simulink model "ModiOmkar_19EE30018_model"  (R2017a)
settings: Solver=FixedStepAuto  StartTime=0.0  StopTime=0.08  FixedStep=1e-7  MaxStep=1e-7  RelTol=1e-6
libraries: powerlib x162, powerlib_meascontrol x12, simulink x12
(part 1 of 2)
settings Model: Creator=Triptendu  LastModifiedBy=HP
settings SFSimCC: SimUseLocalCustomCode=on
settings RTWCC: RTWUseLocalCustomCode=on

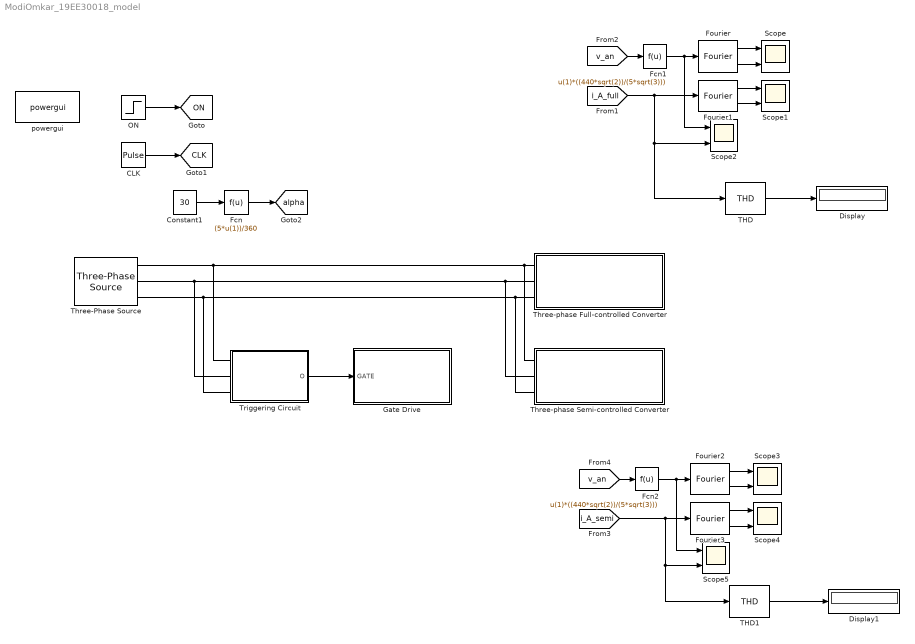
== system ModiOmkar_19EE30018_model ==
  CLK : DiscretePulseGenerator  PulseType=Time based  Period=40e-6  PulseWidth=50
  Constant1 : Constant  Value=30
  Display : Display
  Display1 : Display
  Fcn : Fcn  Expr=(5*u(1))/360
  Fcn1 : Fcn  Expr=u(1)*((440*sqrt(2))/(5*sqrt(3)))
  Fcn2 : Fcn  Expr=u(1)*((440*sqrt(2))/(5*sqrt(3)))
  Fourier{,1..3} (4 alike) : powerlib_meascontrol/Measurements/Fourier  Freq=50  n=1  InInit=[0, 0]  Ts=1e-6
  Gate Drive : Subsystem
  ON : Step  Time=0.002  SampleTime=0
  Scope{,1..5} (6 alike) : Scope  NumInputPorts=2
  THD : powerlib_meascontrol/Measurements/THD  Freq=50  Ts=0
  THD1 : powerlib_meascontrol/Measurements/THD  Freq=50  Ts=0
  Three-Phase Source : powerlib/Electrical Sources/Three-Phase Source  InternalConnection=Y  VoltagePhases=off  Voltage=440  PhaseAngle=0  Voltage_phases=[25e3 25e3 25e3]/sqrt(3)  PhaseAngles_phases=[0 -120 +120]  Frequency=50  NonIdealSource=on  SpecifyImpedance=off  Resistance=0  Inductance=0  ShortCircuitLevel=100e6  BaseVoltage=440  XRratio=7  BusType=swing  Pref=10e3  Qref=0  Prefabc=[10e3, 10e3, 10e3]  Qrefabc=[0, 0, 0]  Qmin=-inf  Qmax=inf
  Three-phase Full-controlled Converter : Subsystem
  Three-phase Semi-controlled Converter : Subsystem
  Triggering Circuit : Subsystem
  powergui : powerlib/powergui  Priority=1  SimulationMode=Discrete  SampleTime=1e-7  frequency=60  Iterations=50  frequencyindice=0  Pbase=100e6  ErrMax=1e-4  UnitsV=kV  UnitsW=MW  buscounter=0  FunctionMessages=off  echomessages=off  EnableUseOfTLC=off  CurrentSourceSwitches=off  DisableSnubberDevices=off  DisableRonSwitches=off  DisableVfSwitches=off  DisplayEquations=off  AutomaticDiscreteSolvers=off  SolverType=Backward Euler  Interpol=off  ExternalGateDelay=off  methode=off  Ts=100  x0status=blocks  SPID=on  SwTol=0  HookPort=off  NonlinearTolerance=1e-4  nMaxIteration=100  ContinueOnMaxIteration=off  RestoreLinks=warning  ResistiveCurrentMeasurement=off  Frange=[0:2:500]  Ylog=off  Xlog=on  ShowGrid=off  save=off  variable=ZData  structure=i_ABC_semi  ZoomFFT=on  StartTime=0.04  cycles=2  DisplayStyle=2  fundamental=50  FreqAxis=off  MaxFrequency=1000  frequencyindicesteady=1  RmsSteady=1  display=off
  tag scope: CLK=global, ON=global, alpha=global
  wires:
  ON/1 -> [ON]
  CLK/1 -> [CLK]
  Constant1/1 -> Fcn/1
  Fcn/1 -> [alpha]
  Triggering Circuit/1(O) -> Gate Drive/1(GATE)
  [i_A_full] -> Scope2/2, THD/1, Fourier1/1
  Fourier/1 -> Scope/1
  Fourier1/1 -> Scope1/1
  [v_an] -> Fcn1/1
  Fcn1/1 -> Scope2/1, Fourier/1
  Fourier/2 -> Scope/2
  Fourier1/2 -> Scope1/2
  [i_A_semi] -> Fourier3/1, THD1/1, Scope5/2
  Fourier2/1 -> Scope3/1
  [v_an] -> Fcn2/1
  Fcn2/1 -> Scope5/1, Fourier2/1
  Fourier3/1 -> Scope4/1
  Fourier2/2 -> Scope3/2
  Fourier3/2 -> Scope4/2
  THD/1 -> Display/1
  THD1/1 -> Display1/1
  connections:
  Triggering Circuit/LConn1 -- Three-phase Semi-controlled Converter/LConn1 -- Three-phase Full-controlled Converter/LConn1 -- Three-Phase Source/RConn1
  Triggering Circuit/LConn2 -- Three-phase Full-controlled Converter/LConn2 -- Three-phase Semi-controlled Converter/LConn2 -- Three-Phase Source/RConn2
  Triggering Circuit/LConn3 -- Three-phase Full-controlled Converter/LConn3 -- Three-phase Semi-controlled Converter/LConn3 -- Three-Phase Source/RConn3

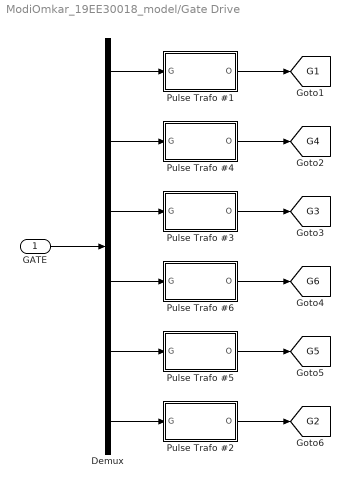
== system ModiOmkar_19EE30018_model/Gate Drive ==
  GATE : Inport
  Demux : Demux  Outputs=6
  Pulse Trafo #1 : Subsystem
  Pulse Trafo #2 : Subsystem
  Pulse Trafo #3 : Subsystem
  Pulse Trafo #4 : Subsystem
  Pulse Trafo #5 : Subsystem
  Pulse Trafo #6 : Subsystem
  tag scope: G1=global, G2=global, G3=global, G4=global, G5=global, G6=global
  wires:
  Demux/6 -> Pulse Trafo #2/1(G)
  Demux/5 -> Pulse Trafo #5/1(G)
  Demux/4 -> Pulse Trafo #6/1(G)
  Demux/3 -> Pulse Trafo #3/1(G)
  Demux/2 -> Pulse Trafo #4/1(G)
  Demux/1 -> Pulse Trafo #1/1(G)
  GATE/1 -> Demux/1
  Pulse Trafo #1/1(O) -> [G1]
  Pulse Trafo #4/1(O) -> [G4]
  Pulse Trafo #3/1(O) -> [G3]
  Pulse Trafo #6/1(O) -> [G6]
  Pulse Trafo #5/1(O) -> [G5]
  Pulse Trafo #2/1(O) -> [G2]

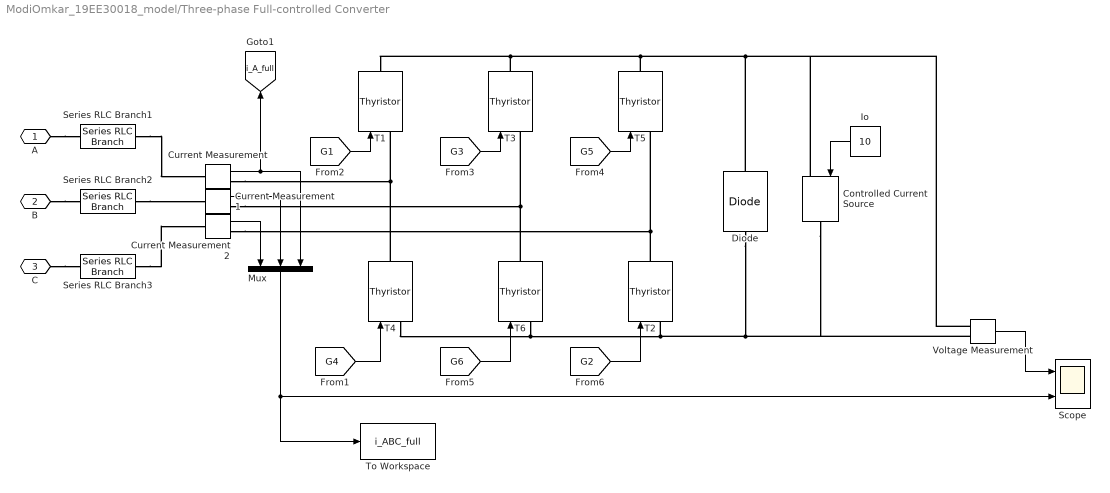
== system ModiOmkar_19EE30018_model/Three-phase Full-controlled Converter ==
  Controlled Current Source : powerlib/Electrical Sources/Controlled Current Source  Initialize=off  Source_Type=DC  Amplitude=0  Phase=0  Frequency=0  Measurements=None
  Current Measurement : powerlib/Measurements/Current Measurement  PhasorSimulation=off  OutputType=Complex  PSBequivalent=0
  Current Measurement1 : powerlib/Measurements/Current Measurement  PhasorSimulation=off  OutputType=Complex  PSBequivalent=0
  Current Measurement2 : powerlib/Measurements/Current Measurement  PhasorSimulation=off  OutputType=Complex  PSBequivalent=0
  Diode : powerlib/Power Electronics/Diode  Ron=1e-6  Lon=0  Vf=0  IC=0  UseSnubber=0  Rs=1e12  Cs=0  Measurements=off
  Io : Constant  Value=10
  Mux : Mux  Inputs=3
  Scope : Scope  NumInputPorts=2
  Series RLC Branch1 : powerlib/Elements/Series RLC Branch  LConnTagsString=__new0  RConnTagsString=__new0  BranchType=R  Resistance=1e-3  Inductance=5e-3  SetiL0=off  InitialCurrent=0  Capacitance=1e-6  Setx0=off  InitialVoltage=0  Measurements=None
  Series RLC Branch2 : powerlib/Elements/Series RLC Branch  LConnTagsString=__new0  RConnTagsString=__new0  BranchType=R  Resistance=1e-3  Inductance=5e-3  SetiL0=off  InitialCurrent=0  Capacitance=1e-6  Setx0=off  InitialVoltage=0  Measurements=None
  Series RLC Branch3 : powerlib/Elements/Series RLC Branch  LConnTagsString=__new0  RConnTagsString=__new0  BranchType=R  Resistance=1e-3  Inductance=5e-3  SetiL0=off  InitialCurrent=0  Capacitance=1e-6  Setx0=off  InitialVoltage=0  Measurements=None
  T{1..6} (6 alike) : powerlib/Power Electronics/Thyristor  Ron=1e-3  Lon=0  Vf=0  IC=0  Rs=1e12  Cs=inf  Measurements=off
  To Workspace : ToWorkspace  VariableName=i_ABC_full  SaveFormat=Structure With Time  SampleTime=-1
  Voltage Measurement : powerlib/Measurements/Voltage Measurement  PhasorSimulation=off  OutputType=Complex  PSBequivalent=0
  A : PMIOPort  Side=Left
  B : PMIOPort  Port=2  Side=Left
  C : PMIOPort  Port=3  Side=Left
  tag scope: i_A_full=global
  wires:
  [G6] -> T6/1
  [G2] -> T2/1
  [G4] -> T4/1
  [G5] -> T5/1
  [G3] -> T3/1
  [G1] -> T1/1
  Voltage Measurement/1 -> Scope/1
  Current Measurement/1 -> Mux/3, [i_A_full]
  Current Measurement1/1 -> Mux/2
  Current Measurement2/1 -> Mux/1
  Io/1 -> Controlled Current Source/1
  Mux/1 -> To Workspace/1, Scope/2
  connections:
  T2/RConn1 -- Current Measurement2/RConn1 -- T5/LConn1
  T5/RConn1 -- Voltage Measurement/LConn1 -- Controlled Current Source/LConn1 -- Diode/RConn1 -- T3/RConn1 -- T1/RConn1
  T6/RConn1 -- Current Measurement1/RConn1 -- T3/LConn1
  T4/RConn1 -- Current Measurement/RConn1 -- T1/LConn1
  C/RConn1 -- Series RLC Branch3/RConn1
  Series RLC Branch1/LConn1 -- Current Measurement/LConn1
  B/RConn1 -- Series RLC Branch2/RConn1
  T4/LConn1 -- T6/LConn1 -- Voltage Measurement/LConn2 -- Controlled Current Source/RConn1 -- Diode/LConn1 -- T2/LConn1
  A/RConn1 -- Series RLC Branch1/RConn1
  Series RLC Branch2/LConn1 -- Current Measurement1/LConn1
  Series RLC Branch3/LConn1 -- Current Measurement2/LConn1

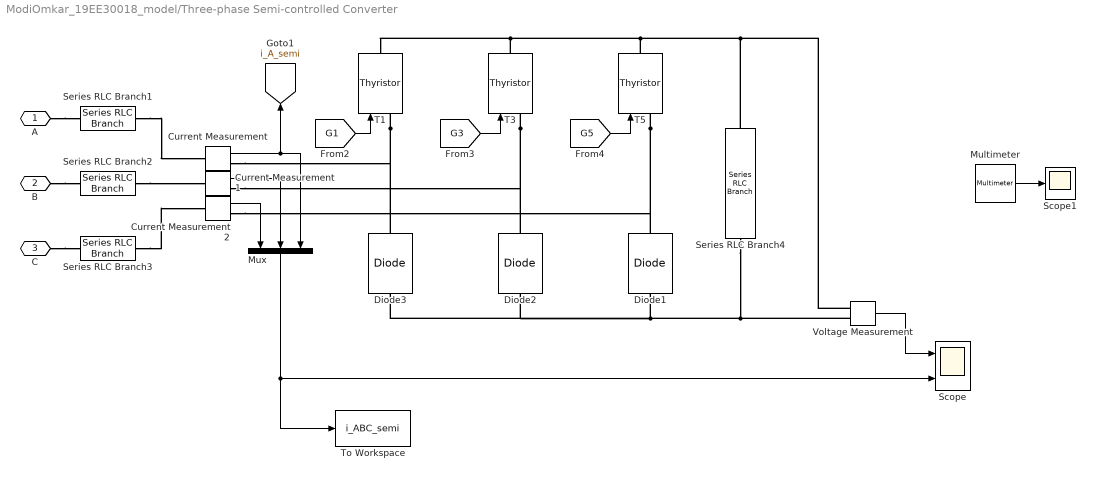
== system ModiOmkar_19EE30018_model/Three-phase Semi-controlled Converter ==
  Current Measurement : powerlib/Measurements/Current Measurement  PhasorSimulation=off  OutputType=Complex  PSBequivalent=0
  Current Measurement1 : powerlib/Measurements/Current Measurement  PhasorSimulation=off  OutputType=Complex  PSBequivalent=0
  Current Measurement2 : powerlib/Measurements/Current Measurement  PhasorSimulation=off  OutputType=Complex  PSBequivalent=0
  Diode1 : powerlib/Power Electronics/Diode  Ron=1e-3  Lon=0  Vf=0  IC=0  UseSnubber=0  Rs=1e12  Cs=inf  Measurements=off
  Diode2 : powerlib/Power Electronics/Diode  Ron=1e-3  Lon=0  Vf=0  IC=0  UseSnubber=0  Rs=1e12  Cs=inf  Measurements=off
  Diode3 : powerlib/Power Electronics/Diode  Ron=1e-3  Lon=0  Vf=0  IC=0  UseSnubber=0  Rs=1e12  Cs=inf  Measurements=off
  Multimeter : powerlib/Measurements/Multimeter  PhasorSimulation=off  OutputType=Complex  sel=1  L=1  Gain=1  yselected={'Ib: Three-phase Semi-controlled Converter/Series RLC Branch4'};  PSBOutputType=1  PSBequivalent=0  AxesSetting=[0,0.1,-100,100]  Display=0  SavedBlockNames=-11
  Mux : Mux  Inputs=3
  Scope : Scope  NumInputPorts=2
  Scope1 : Scope
  Series RLC Branch1 : powerlib/Elements/Series RLC Branch  LConnTagsString=__new0  RConnTagsString=__new0  BranchType=R  Resistance=1e-3  Inductance=5e-3  SetiL0=off  InitialCurrent=0  Capacitance=1e-6  Setx0=off  InitialVoltage=0  Measurements=None
  Series RLC Branch2 : powerlib/Elements/Series RLC Branch  LConnTagsString=__new0  RConnTagsString=__new0  BranchType=R  Resistance=1e-3  Inductance=5e-3  SetiL0=off  InitialCurrent=0  Capacitance=1e-6  Setx0=off  InitialVoltage=0  Measurements=None
  Series RLC Branch3 : powerlib/Elements/Series RLC Branch  LConnTagsString=__new0  RConnTagsString=__new0  BranchType=R  Resistance=1e-3  Inductance=5e-3  SetiL0=off  InitialCurrent=0  Capacitance=1e-6  Setx0=off  InitialVoltage=0  Measurements=None
  Series RLC Branch4 : powerlib/Elements/Series RLC Branch  LConnTagsString=__new0  RConnTagsString=__new0  BranchType=RL  Resistance=50.7188  Inductance=100e-3  SetiL0=off  InitialCurrent=0  Capacitance=1e-6  Setx0=off  InitialVoltage=0  Measurements=Branch current
  T1 : powerlib/Power Electronics/Thyristor  Ron=1e-3  Lon=0  Vf=0  IC=0  Rs=1e12  Cs=inf  Measurements=off
  T3 : powerlib/Power Electronics/Thyristor  Ron=1e-3  Lon=0  Vf=0  IC=0  Rs=1e12  Cs=inf  Measurements=off
  T5 : powerlib/Power Electronics/Thyristor  Ron=1e-3  Lon=0  Vf=0  IC=0  Rs=1e12  Cs=inf  Measurements=off
  To Workspace : ToWorkspace  VariableName=i_ABC_semi  SaveFormat=Structure With Time  SampleTime=-1
  Voltage Measurement : powerlib/Measurements/Voltage Measurement  PhasorSimulation=off  OutputType=Complex  PSBequivalent=0
  A : PMIOPort  Side=Left
  B : PMIOPort  Port=2  Side=Left
  C : PMIOPort  Port=3  Side=Left
  tag scope: i_A_semi=global
  wires:
  Current Measurement2/1 -> Mux/1
  Current Measurement1/1 -> Mux/2
  Current Measurement/1 -> [i_A_semi], Mux/3
  Voltage Measurement/1 -> Scope/1
  [G1] -> T1/1
  [G3] -> T3/1
  [G5] -> T5/1
  Multimeter/1 -> Scope1/1
  Mux/1 -> To Workspace/1, Scope/2
  connections:
  Series RLC Branch3/LConn1 -- Current Measurement2/LConn1
  Series RLC Branch2/LConn1 -- Current Measurement1/LConn1
  A/RConn1 -- Series RLC Branch1/RConn1
  Voltage Measurement/LConn2 -- Series RLC Branch4/LConn1 -- Diode2/LConn1 -- Diode3/LConn1 -- Diode1/LConn1
  B/RConn1 -- Series RLC Branch2/RConn1
  Series RLC Branch1/LConn1 -- Current Measurement/LConn1
  C/RConn1 -- Series RLC Branch3/RConn1
  T1/LConn1 -- Diode3/RConn1 -- Current Measurement/RConn1
  T3/LConn1 -- Diode2/RConn1 -- Current Measurement1/RConn1
  Voltage Measurement/LConn1 -- Series RLC Branch4/RConn1 -- T1/RConn1 -- T3/RConn1 -- T5/RConn1
  T5/LConn1 -- Diode1/RConn1 -- Current Measurement2/RConn1

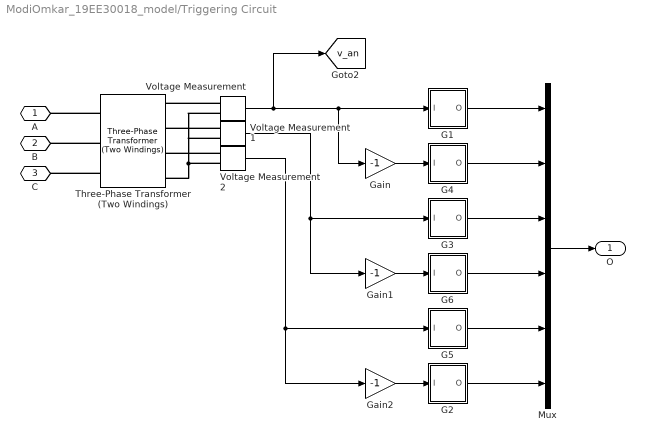
== system ModiOmkar_19EE30018_model/Triggering Circuit ==
  G1 : Subsystem
  G2 : Subsystem
  G3 : Subsystem
  G4 : Subsystem
  G5 : Subsystem
  G6 : Subsystem
  Gain : Gain  Gain=-1
  Gain1 : Gain  Gain=-1
  Gain2 : Gain  Gain=-1
  Mux : Mux  Inputs=6
  Three-Phase Transformer (Two Windings) : powerlib/Elements/Three-Phase Transformer (Two Windings)  Winding1Connection=Y  Winding2Connection=Yn  CoreType=Three single-phase transformers  SetSaturation=off  Hysteresis=off  DataFile='hysteresis'  SetInitialFlux=off  Measurements=None  UNITS=SI  NominalPower=[ 100 , 50 ]  Winding1=[440*sqrt(2) 0 0]  Winding2=[5*sqrt(3) 0 0]  Rm=1e6  Lm=1e6  L0=0.5  Saturation=[0 0;0.00044536 1.3723;0.18557 1.7382]  InitialFluxes=[ 0.8 , -0.8 , 0.7 ]  BreakLoop=off  DiscreteSolver=Trapezoidal iterative  DataType=on  TransfoNumber=1
  Voltage Measurement : powerlib/Measurements/Voltage Measurement  PhasorSimulation=off  OutputType=Complex  PSBequivalent=0
  Voltage Measurement1 : powerlib/Measurements/Voltage Measurement  PhasorSimulation=off  OutputType=Complex  PSBequivalent=0
  Voltage Measurement2 : powerlib/Measurements/Voltage Measurement  PhasorSimulation=off  OutputType=Complex  PSBequivalent=0
  A : PMIOPort  Side=Left
  B : PMIOPort  Port=2  Side=Left
  C : PMIOPort  Port=3  Side=Left
  O : Outport
  tag scope: v_an=global
  wires:
  G1/1(O) -> Mux/1
  Gain/1 -> G4/1(I)
  Gain1/1 -> G6/1(I)
  G5/1(O) -> Mux/5
  Voltage Measurement1/1 -> G3/1(I), Gain1/1
  Voltage Measurement2/1 -> G5/1(I), Gain2/1
  Gain2/1 -> G2/1(I)
  Voltage Measurement/1 -> [v_an], G1/1(I), Gain/1
  G3/1(O) -> Mux/3
  G4/1(O) -> Mux/2
  G2/1(O) -> Mux/6
  G6/1(O) -> Mux/4
  Mux/1 -> O/1
  connections:
  Voltage Measurement2/LConn2 -- Voltage Measurement1/LConn2 -- Voltage Measurement/LConn2 -- Three-Phase Transformer (Two Windings)/RConn4
  Voltage Measurement2/LConn1 -- Three-Phase Transformer (Two Windings)/RConn3
  Voltage Measurement/LConn1 -- Three-Phase Transformer (Two Windings)/RConn1
  Three-Phase Transformer (Two Windings)/LConn2 -- B/RConn1
  Voltage Measurement1/LConn1 -- Three-Phase Transformer (Two Windings)/RConn2
  Three-Phase Transformer (Two Windings)/LConn1 -- A/RConn1
  Three-Phase Transformer (Two Windings)/LConn3 -- C/RConn1

== system ModiOmkar_19EE30018_model/Gate Drive/Pulse Trafo #1 ==
  G : Inport
  D1 : powerlib/Power Electronics/Diode  Ron=0.001  Lon=0  Vf=0.7  IC=0  UseSnubber=off  Rs=inf  Cs=0  Measurements=off
  Ground5 : powerlib/Elements/Ground  LConnTagsString=a
  Ground6 : powerlib/Elements/Ground  LConnTagsString=a
  Mosfet : powerlib/Power Electronics/Mosfet  Ron=0.1  Lon=0  Rd=0.01  Vfd=0  IC=0  Rs=1e5  Cs=inf  Measurements=off
  R : powerlib/Elements/Series RLC Branch  LConnTagsString=__new0  RConnTagsString=__new0  BranchType=R  Resistance=10  Inductance=60e-3  SetiL0=off  InitialCurrent=0  Capacitance=1e-6  Setx0=off  InitialVoltage=0  Measurements=None
  R (for simulation) : powerlib/Elements/Series RLC Branch  LConnTagsString=__new0  RConnTagsString=__new0  BranchType=R  Resistance=1e6  Inductance=60e-3  SetiL0=off  InitialCurrent=0  Capacitance=1e-6  Setx0=off  InitialVoltage=0  Measurements=None
  Subsystem : Subsystem
  Vcc : powerlib/Electrical Sources/DC Voltage Source  Amplitude=20  Measurements=None
  Zener Diode : Subsystem  mask(Zener Diode){Vz=40, Rzt=10, Rzk=400, Izm=5, Vf=0.7, Ron=1e-3}
      mask prompts: Vz "Zener Voltage Vz (V)"; Rzt "Dynamic Impedance Zzt (ohms)"; Rzk "Knee Impedance Zzk (ohms)"; Izm "Maximum Continuous Current Izm (A)"; Vf "Forward Voltage Drop Vf (V)"; Ron "On Resistance Ron (ohms)"
      mask help:
      | Implements a zener diode block.
      | Use values from standard datasheets to populate block dialog
  pulse transformer : powerlib/Elements/Linear Transformer  UNITS=SI  NominalPower=[0.5 500e3 ]  winding1=[20 0.08 2e-6]  winding2=[20 0.08 2e-6]  ThreeWindings=off  winding3=[5 0.8 20e-6]  RmLm=[400 5e-3]  Measurements=None  DataType=on
  O : Outport
  wires:
  Subsystem/1(O) -> O/1
  G/1 -> Mosfet/1
  connections:
  Subsystem/LConn2 -- pulse transformer/RConn2
  pulse transformer/RConn1 -- Subsystem/LConn1
  D1/LConn1 -- Zener Diode/RConn1 -- R (for simulation)/RConn1
  D1/RConn1 -- Vcc/RConn1 -- R/LConn1
  Ground5/LConn1 -- Vcc/LConn1
  Ground6/LConn1 -- Mosfet/RConn1
  Mosfet/LConn1 -- Zener Diode/LConn1 -- R (for simulation)/LConn1 -- pulse transformer/LConn2
  R/RConn1 -- pulse transformer/LConn1

== system ModiOmkar_19EE30018_model/Gate Drive/Pulse Trafo #2 ==
  G : Inport
  D1 : powerlib/Power Electronics/Diode  Ron=0.001  Lon=0  Vf=0.7  IC=0  UseSnubber=off  Rs=inf  Cs=0  Measurements=off
  Ground5 : powerlib/Elements/Ground  LConnTagsString=a
  Ground6 : powerlib/Elements/Ground  LConnTagsString=a
  Mosfet : powerlib/Power Electronics/Mosfet  Ron=0.1  Lon=0  Rd=0.01  Vfd=0  IC=0  Rs=1e5  Cs=inf  Measurements=off
  R : powerlib/Elements/Series RLC Branch  LConnTagsString=__new0  RConnTagsString=__new0  BranchType=R  Resistance=10  Inductance=60e-3  SetiL0=off  InitialCurrent=0  Capacitance=1e-6  Setx0=off  InitialVoltage=0  Measurements=None
  R (for simulation) : powerlib/Elements/Series RLC Branch  LConnTagsString=__new0  RConnTagsString=__new0  BranchType=R  Resistance=1e6  Inductance=60e-3  SetiL0=off  InitialCurrent=0  Capacitance=1e-6  Setx0=off  InitialVoltage=0  Measurements=None
  Subsystem : Subsystem
  Vcc : powerlib/Electrical Sources/DC Voltage Source  Amplitude=20  Measurements=None
  Zener Diode : Subsystem  mask(Zener Diode){Vz=40, Rzt=10, Rzk=400, Izm=5, Vf=0.7, Ron=1e-3}
      mask prompts: Vz "Zener Voltage Vz (V)"; Rzt "Dynamic Impedance Zzt (ohms)"; Rzk "Knee Impedance Zzk (ohms)"; Izm "Maximum Continuous Current Izm (A)"; Vf "Forward Voltage Drop Vf (V)"; Ron "On Resistance Ron (ohms)"
      mask help:
      | Implements a zener diode block.
      | Use values from standard datasheets to populate block dialog
  pulse transformer : powerlib/Elements/Linear Transformer  UNITS=SI  NominalPower=[0.5 500e3 ]  winding1=[20 0.08 2e-6]  winding2=[20 0.08 2e-6]  ThreeWindings=off  winding3=[5 0.8 20e-6]  RmLm=[400 5e-3]  Measurements=None  DataType=on
  O : Outport
  wires:
  G/1 -> Mosfet/1
  Subsystem/1(O) -> O/1
  connections:
  R/RConn1 -- pulse transformer/LConn1
  pulse transformer/LConn2 -- R (for simulation)/LConn1 -- Zener Diode/LConn1 -- Mosfet/LConn1
  Ground6/LConn1 -- Mosfet/RConn1
  Ground5/LConn1 -- Vcc/LConn1
  Vcc/RConn1 -- R/LConn1 -- D1/RConn1
  R (for simulation)/RConn1 -- Zener Diode/RConn1 -- D1/LConn1
  pulse transformer/RConn1 -- Subsystem/LConn1
  Subsystem/LConn2 -- pulse transformer/RConn2

== system ModiOmkar_19EE30018_model/Gate Drive/Pulse Trafo #3 ==
  G : Inport
  D1 : powerlib/Power Electronics/Diode  Ron=0.001  Lon=0  Vf=0.7  IC=0  UseSnubber=off  Rs=inf  Cs=0  Measurements=off
  Ground5 : powerlib/Elements/Ground  LConnTagsString=a
  Ground6 : powerlib/Elements/Ground  LConnTagsString=a
  Mosfet : powerlib/Power Electronics/Mosfet  Ron=0.1  Lon=0  Rd=0.01  Vfd=0  IC=0  Rs=1e5  Cs=inf  Measurements=off
  R : powerlib/Elements/Series RLC Branch  LConnTagsString=__new0  RConnTagsString=__new0  BranchType=R  Resistance=10  Inductance=60e-3  SetiL0=off  InitialCurrent=0  Capacitance=1e-6  Setx0=off  InitialVoltage=0  Measurements=None
  R (for simulation) : powerlib/Elements/Series RLC Branch  LConnTagsString=__new0  RConnTagsString=__new0  BranchType=R  Resistance=1e6  Inductance=60e-3  SetiL0=off  InitialCurrent=0  Capacitance=1e-6  Setx0=off  InitialVoltage=0  Measurements=None
  Subsystem : Subsystem
  Vcc : powerlib/Electrical Sources/DC Voltage Source  Amplitude=20  Measurements=None
  Zener Diode : Subsystem  mask(Zener Diode){Vz=40, Rzt=10, Rzk=400, Izm=5, Vf=0.7, Ron=1e-3}
      mask prompts: Vz "Zener Voltage Vz (V)"; Rzt "Dynamic Impedance Zzt (ohms)"; Rzk "Knee Impedance Zzk (ohms)"; Izm "Maximum Continuous Current Izm (A)"; Vf "Forward Voltage Drop Vf (V)"; Ron "On Resistance Ron (ohms)"
      mask help:
      | Implements a zener diode block.
      | Use values from standard datasheets to populate block dialog
  pulse transformer : powerlib/Elements/Linear Transformer  UNITS=SI  NominalPower=[0.5 500e3 ]  winding1=[20 0.08 2e-6]  winding2=[20 0.08 2e-6]  ThreeWindings=off  winding3=[5 0.8 20e-6]  RmLm=[400 5e-3]  Measurements=None  DataType=on
  O : Outport
  wires:
  Subsystem/1(O) -> O/1
  G/1 -> Mosfet/1
  connections:
  Subsystem/LConn2 -- pulse transformer/RConn2
  pulse transformer/RConn1 -- Subsystem/LConn1
  D1/LConn1 -- Zener Diode/RConn1 -- R (for simulation)/RConn1
  D1/RConn1 -- R/LConn1 -- Vcc/RConn1
  Ground5/LConn1 -- Vcc/LConn1
  Ground6/LConn1 -- Mosfet/RConn1
  Mosfet/LConn1 -- Zener Diode/LConn1 -- R (for simulation)/LConn1 -- pulse transformer/LConn2
  R/RConn1 -- pulse transformer/LConn1

== system ModiOmkar_19EE30018_model/Gate Drive/Pulse Trafo #4 ==
  G : Inport
  D1 : powerlib/Power Electronics/Diode  Ron=0.001  Lon=0  Vf=0.7  IC=0  UseSnubber=off  Rs=inf  Cs=0  Measurements=off
  Ground5 : powerlib/Elements/Ground  LConnTagsString=a
  Ground6 : powerlib/Elements/Ground  LConnTagsString=a
  Mosfet : powerlib/Power Electronics/Mosfet  Ron=0.1  Lon=0  Rd=0.01  Vfd=0  IC=0  Rs=1e5  Cs=inf  Measurements=off
  R : powerlib/Elements/Series RLC Branch  LConnTagsString=__new0  RConnTagsString=__new0  BranchType=R  Resistance=10  Inductance=60e-3  SetiL0=off  InitialCurrent=0  Capacitance=1e-6  Setx0=off  InitialVoltage=0  Measurements=None
  R (for simulation) : powerlib/Elements/Series RLC Branch  LConnTagsString=__new0  RConnTagsString=__new0  BranchType=R  Resistance=1e6  Inductance=60e-3  SetiL0=off  InitialCurrent=0  Capacitance=1e-6  Setx0=off  InitialVoltage=0  Measurements=None
  Subsystem : Subsystem
  Vcc : powerlib/Electrical Sources/DC Voltage Source  Amplitude=20  Measurements=None
  Zener Diode : Subsystem  mask(Zener Diode){Vz=40, Rzt=10, Rzk=400, Izm=5, Vf=0.7, Ron=1e-3}
      mask prompts: Vz "Zener Voltage Vz (V)"; Rzt "Dynamic Impedance Zzt (ohms)"; Rzk "Knee Impedance Zzk (ohms)"; Izm "Maximum Continuous Current Izm (A)"; Vf "Forward Voltage Drop Vf (V)"; Ron "On Resistance Ron (ohms)"
      mask help:
      | Implements a zener diode block.
      | Use values from standard datasheets to populate block dialog
  pulse transformer : powerlib/Elements/Linear Transformer  UNITS=SI  NominalPower=[0.5 500e3 ]  winding1=[20 0.08 2e-6]  winding2=[20 0.08 2e-6]  ThreeWindings=off  winding3=[5 0.8 20e-6]  RmLm=[400 5e-3]  Measurements=None  DataType=on
  O : Outport
  wires:
  G/1 -> Mosfet/1
  Subsystem/1(O) -> O/1
  connections:
  R/RConn1 -- pulse transformer/LConn1
  pulse transformer/LConn2 -- R (for simulation)/LConn1 -- Zener Diode/LConn1 -- Mosfet/LConn1
  Ground6/LConn1 -- Mosfet/RConn1
  Ground5/LConn1 -- Vcc/LConn1
  Vcc/RConn1 -- R/LConn1 -- D1/RConn1
  R (for simulation)/RConn1 -- Zener Diode/RConn1 -- D1/LConn1
  pulse transformer/RConn1 -- Subsystem/LConn1
  Subsystem/LConn2 -- pulse transformer/RConn2

== system ModiOmkar_19EE30018_model/Gate Drive/Pulse Trafo #5 ==
  G : Inport
  D1 : powerlib/Power Electronics/Diode  Ron=0.001  Lon=0  Vf=0.7  IC=0  UseSnubber=off  Rs=inf  Cs=0  Measurements=off
  Ground5 : powerlib/Elements/Ground  LConnTagsString=a
  Ground6 : powerlib/Elements/Ground  LConnTagsString=a
  Mosfet : powerlib/Power Electronics/Mosfet  Ron=0.1  Lon=0  Rd=0.01  Vfd=0  IC=0  Rs=1e5  Cs=inf  Measurements=off
  R : powerlib/Elements/Series RLC Branch  LConnTagsString=__new0  RConnTagsString=__new0  BranchType=R  Resistance=10  Inductance=60e-3  SetiL0=off  InitialCurrent=0  Capacitance=1e-6  Setx0=off  InitialVoltage=0  Measurements=None
  R (for simulation) : powerlib/Elements/Series RLC Branch  LConnTagsString=__new0  RConnTagsString=__new0  BranchType=R  Resistance=1e6  Inductance=60e-3  SetiL0=off  InitialCurrent=0  Capacitance=1e-6  Setx0=off  InitialVoltage=0  Measurements=None
  Subsystem : Subsystem
  Vcc : powerlib/Electrical Sources/DC Voltage Source  Amplitude=20  Measurements=None
  Zener Diode : Subsystem  mask(Zener Diode){Vz=40, Rzt=10, Rzk=400, Izm=5, Vf=0.7, Ron=1e-3}
      mask prompts: Vz "Zener Voltage Vz (V)"; Rzt "Dynamic Impedance Zzt (ohms)"; Rzk "Knee Impedance Zzk (ohms)"; Izm "Maximum Continuous Current Izm (A)"; Vf "Forward Voltage Drop Vf (V)"; Ron "On Resistance Ron (ohms)"
      mask help:
      | Implements a zener diode block.
      | Use values from standard datasheets to populate block dialog
  pulse transformer : powerlib/Elements/Linear Transformer  UNITS=SI  NominalPower=[0.5 500e3 ]  winding1=[20 0.08 2e-6]  winding2=[20 0.08 2e-6]  ThreeWindings=off  winding3=[5 0.8 20e-6]  RmLm=[400 5e-3]  Measurements=None  DataType=on
  O : Outport
  wires:
  G/1 -> Mosfet/1
  Subsystem/1(O) -> O/1
  connections:
  R/RConn1 -- pulse transformer/LConn1
  pulse transformer/LConn2 -- R (for simulation)/LConn1 -- Zener Diode/LConn1 -- Mosfet/LConn1
  Ground6/LConn1 -- Mosfet/RConn1
  Ground5/LConn1 -- Vcc/LConn1
  Vcc/RConn1 -- R/LConn1 -- D1/RConn1
  R (for simulation)/RConn1 -- Zener Diode/RConn1 -- D1/LConn1
  pulse transformer/RConn1 -- Subsystem/LConn1
  Subsystem/LConn2 -- pulse transformer/RConn2

== system ModiOmkar_19EE30018_model/Gate Drive/Pulse Trafo #6 ==
  G : Inport
  D1 : powerlib/Power Electronics/Diode  Ron=0.001  Lon=0  Vf=0.7  IC=0  UseSnubber=off  Rs=inf  Cs=0  Measurements=off
  Ground5 : powerlib/Elements/Ground  LConnTagsString=a
  Ground6 : powerlib/Elements/Ground  LConnTagsString=a
  Mosfet : powerlib/Power Electronics/Mosfet  Ron=0.1  Lon=0  Rd=0.01  Vfd=0  IC=0  Rs=1e5  Cs=inf  Measurements=off
  R : powerlib/Elements/Series RLC Branch  LConnTagsString=__new0  RConnTagsString=__new0  BranchType=R  Resistance=10  Inductance=60e-3  SetiL0=off  InitialCurrent=0  Capacitance=1e-6  Setx0=off  InitialVoltage=0  Measurements=None
  R (for simulation) : powerlib/Elements/Series RLC Branch  LConnTagsString=__new0  RConnTagsString=__new0  BranchType=R  Resistance=1e6  Inductance=60e-3  SetiL0=off  InitialCurrent=0  Capacitance=1e-6  Setx0=off  InitialVoltage=0  Measurements=None
  Subsystem : Subsystem
  Vcc : powerlib/Electrical Sources/DC Voltage Source  Amplitude=20  Measurements=None
  Zener Diode : Subsystem  mask(Zener Diode){Vz=40, Rzt=10, Rzk=400, Izm=5, Vf=0.7, Ron=1e-3}
      mask prompts: Vz "Zener Voltage Vz (V)"; Rzt "Dynamic Impedance Zzt (ohms)"; Rzk "Knee Impedance Zzk (ohms)"; Izm "Maximum Continuous Current Izm (A)"; Vf "Forward Voltage Drop Vf (V)"; Ron "On Resistance Ron (ohms)"
      mask help:
      | Implements a zener diode block.
      | Use values from standard datasheets to populate block dialog
  pulse transformer : powerlib/Elements/Linear Transformer  UNITS=SI  NominalPower=[0.5 500e3 ]  winding1=[20 0.08 2e-6]  winding2=[20 0.08 2e-6]  ThreeWindings=off  winding3=[5 0.8 20e-6]  RmLm=[400 5e-3]  Measurements=None  DataType=on
  O : Outport
  wires:
  Subsystem/1(O) -> O/1
  G/1 -> Mosfet/1
  connections:
  Subsystem/LConn2 -- pulse transformer/RConn2
  pulse transformer/RConn1 -- Subsystem/LConn1
  D1/LConn1 -- Zener Diode/RConn1 -- R (for simulation)/RConn1
  D1/RConn1 -- R/LConn1 -- Vcc/RConn1
  Ground5/LConn1 -- Vcc/LConn1
  Ground6/LConn1 -- Mosfet/RConn1
  Mosfet/LConn1 -- Zener Diode/LConn1 -- R (for simulation)/LConn1 -- pulse transformer/LConn2
  R/RConn1 -- pulse transformer/LConn1

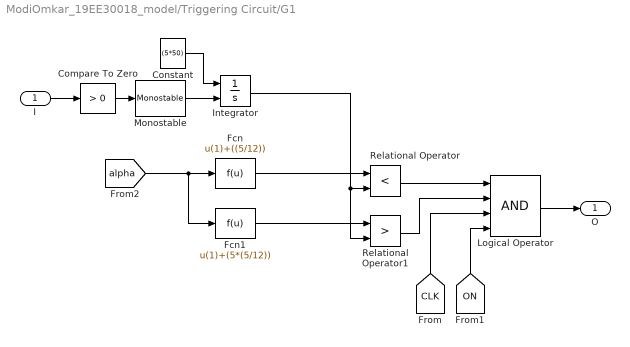
== system ModiOmkar_19EE30018_model/Triggering Circuit/G1 ==
  I : Inport
  Compare To Zero : simulink/Logic and Bit Operations/Compare To Zero  relop=>  OutDataTypeStr=boolean
  Constant : Constant  Value=(5*50)
  Fcn : Fcn  Expr=u(1)+((5/12))
  Fcn1 : Fcn  Expr=u(1)+(5*(5/12))
  Integrator : Integrator  ExternalReset=rising
  Logical Operator : Logic  Inputs=4  AllPortsSameDT=off  OutDataTypeStr=boolean
  Monostable : powerlib_meascontrol/Logic/Monostable  EdgeDetect=Rising  PulseDuration=10e-6  ic=0  Ts=1e-6
      settings: SourceProductBaseCode=PS
  Relational Operator : RelationalOperator  Operator=<  OutDataTypeStr=boolean  RndMeth=Simplest
  Relational Operator1 : RelationalOperator  Operator=>  OutDataTypeStr=boolean  RndMeth=Simplest
  O : Outport
  wires:
  [CLK] -> Logical Operator/3
  Relational Operator1/1 -> Logical Operator/2
  Compare To Zero/1 -> Monostable/1
  Relational Operator/1 -> Logical Operator/1
  [alpha] -> Fcn1/1, Fcn/1
  [ON] -> Logical Operator/4
  Fcn1/1 -> Relational Operator1/1
  Fcn/1 -> Relational Operator/1
  Constant/1 -> Integrator/1
  Monostable/1 -> Integrator/2
  I/1 -> Compare To Zero/1
  Logical Operator/1 -> O/1
  Integrator/1 -> Relational Operator1/2, Relational Operator/2

== system ModiOmkar_19EE30018_model/Triggering Circuit/G2 ==
  I : Inport
  Compare To Zero : simulink/Logic and Bit Operations/Compare To Zero  relop=>  OutDataTypeStr=boolean
  Constant : Constant  Value=(5*50)
  Fcn : Fcn  Expr=u(1)+(5*(1/12))
  Fcn1 : Fcn  Expr=u(1)+(5*(5/12))
  Integrator : Integrator  ExternalReset=rising
  Logical Operator : Logic  Inputs=4  AllPortsSameDT=off  OutDataTypeStr=boolean
  Monostable : powerlib_meascontrol/Logic/Monostable  EdgeDetect=Rising  PulseDuration=10e-6  ic=0  Ts=1e-6
      settings: SourceProductBaseCode=PS
  Relational Operator : RelationalOperator  Operator=<  OutDataTypeStr=boolean  RndMeth=Simplest
  Relational Operator1 : RelationalOperator  Operator=>  OutDataTypeStr=boolean  RndMeth=Simplest
  O : Outport
  wires:
  Integrator/1 -> Relational Operator/2, Relational Operator1/2
  Logical Operator/1 -> O/1
  I/1 -> Compare To Zero/1
  Monostable/1 -> Integrator/2
  Constant/1 -> Integrator/1
  Fcn/1 -> Relational Operator/1
  Fcn1/1 -> Relational Operator1/1
  [ON] -> Logical Operator/4
  [alpha] -> Fcn/1, Fcn1/1
  Relational Operator/1 -> Logical Operator/1
  Compare To Zero/1 -> Monostable/1
  Relational Operator1/1 -> Logical Operator/2
  [CLK] -> Logical Operator/3

== system ModiOmkar_19EE30018_model/Triggering Circuit/G3 ==
  I : Inport
  Compare To Zero : simulink/Logic and Bit Operations/Compare To Zero  relop=>  OutDataTypeStr=boolean
  Constant : Constant  Value=(5*50)
  Fcn : Fcn  Expr=u(1)+(5*(1/12))
  Fcn1 : Fcn  Expr=u(1)+(5*(5/12))
  Integrator : Integrator  ExternalReset=rising
  Logical Operator : Logic  Inputs=4  AllPortsSameDT=off  OutDataTypeStr=boolean
  Monostable : powerlib_meascontrol/Logic/Monostable  EdgeDetect=Rising  PulseDuration=10e-6  ic=0  Ts=1e-6
      settings: SourceProductBaseCode=PS
  Relational Operator : RelationalOperator  Operator=<  OutDataTypeStr=boolean  RndMeth=Simplest
  Relational Operator1 : RelationalOperator  Operator=>  OutDataTypeStr=boolean  RndMeth=Simplest
  O : Outport
  wires:
  [CLK] -> Logical Operator/3
  Relational Operator1/1 -> Logical Operator/2
  Compare To Zero/1 -> Monostable/1
  Relational Operator/1 -> Logical Operator/1
  [alpha] -> Fcn1/1, Fcn/1
  [ON] -> Logical Operator/4
  Fcn1/1 -> Relational Operator1/1
  Fcn/1 -> Relational Operator/1
  Constant/1 -> Integrator/1
  Monostable/1 -> Integrator/2
  I/1 -> Compare To Zero/1
  Logical Operator/1 -> O/1
  Integrator/1 -> Relational Operator1/2, Relational Operator/2

== system ModiOmkar_19EE30018_model/Triggering Circuit/G4 ==
  I : Inport
  Compare To Zero : simulink/Logic and Bit Operations/Compare To Zero  relop=>  OutDataTypeStr=boolean
  Constant : Constant  Value=(5*50)
  Fcn : Fcn  Expr=u(1)+(5*(1/12))
  Fcn1 : Fcn  Expr=u(1)+(5*(5/12))
  Integrator : Integrator  ExternalReset=rising
  Logical Operator : Logic  Inputs=4  AllPortsSameDT=off  OutDataTypeStr=boolean
  Monostable : powerlib_meascontrol/Logic/Monostable  EdgeDetect=Rising  PulseDuration=10e-6  ic=0  Ts=1e-6
      settings: SourceProductBaseCode=PS
  Relational Operator : RelationalOperator  Operator=<  OutDataTypeStr=boolean  RndMeth=Simplest
  Relational Operator1 : RelationalOperator  Operator=>  OutDataTypeStr=boolean  RndMeth=Simplest
  O : Outport
  wires:
  Integrator/1 -> Relational Operator/2, Relational Operator1/2
  Logical Operator/1 -> O/1
  I/1 -> Compare To Zero/1
  Monostable/1 -> Integrator/2
  Constant/1 -> Integrator/1
  Fcn/1 -> Relational Operator/1
  Fcn1/1 -> Relational Operator1/1
  [ON] -> Logical Operator/4
  [alpha] -> Fcn/1, Fcn1/1
  Relational Operator/1 -> Logical Operator/1
  Compare To Zero/1 -> Monostable/1
  Relational Operator1/1 -> Logical Operator/2
  [CLK] -> Logical Operator/3

== system ModiOmkar_19EE30018_model/Triggering Circuit/G5 ==
  I : Inport
  Compare To Zero : simulink/Logic and Bit Operations/Compare To Zero  relop=>  OutDataTypeStr=boolean
  Constant : Constant  Value=(5*50)
  Fcn : Fcn  Expr=u(1)+(5*(1/12))
  Fcn1 : Fcn  Expr=u(1)+(5*(5/12))
  Integrator : Integrator  ExternalReset=rising
  Logical Operator : Logic  Inputs=4  AllPortsSameDT=off  OutDataTypeStr=boolean
  Monostable : powerlib_meascontrol/Logic/Monostable  EdgeDetect=Rising  PulseDuration=10e-6  ic=0  Ts=1e-6
      settings: SourceProductBaseCode=PS
  Relational Operator : RelationalOperator  Operator=<  OutDataTypeStr=boolean  RndMeth=Simplest
  Relational Operator1 : RelationalOperator  Operator=>  OutDataTypeStr=boolean  RndMeth=Simplest
  O : Outport
  wires:
  [CLK] -> Logical Operator/3
  Relational Operator1/1 -> Logical Operator/2
  Compare To Zero/1 -> Monostable/1
  Relational Operator/1 -> Logical Operator/1
  [alpha] -> Fcn1/1, Fcn/1
  [ON] -> Logical Operator/4
  Fcn1/1 -> Relational Operator1/1
  Fcn/1 -> Relational Operator/1
  Constant/1 -> Integrator/1
  Monostable/1 -> Integrator/2
  I/1 -> Compare To Zero/1
  Logical Operator/1 -> O/1
  Integrator/1 -> Relational Operator1/2, Relational Operator/2

== system ModiOmkar_19EE30018_model/Triggering Circuit/G6 ==
  I : Inport
  Compare To Zero : simulink/Logic and Bit Operations/Compare To Zero  relop=>  OutDataTypeStr=boolean
  Constant : Constant  Value=(5*50)
  Fcn : Fcn  Expr=u(1)+(5*(1/12))
  Fcn1 : Fcn  Expr=u(1)+(5*(5/12))
  Integrator : Integrator  ExternalReset=rising
  Logical Operator : Logic  Inputs=4  AllPortsSameDT=off  OutDataTypeStr=boolean
  Monostable : powerlib_meascontrol/Logic/Monostable  EdgeDetect=Rising  PulseDuration=10e-6  ic=0  Ts=1e-6
      settings: SourceProductBaseCode=PS
  Relational Operator : RelationalOperator  Operator=<  OutDataTypeStr=boolean  RndMeth=Simplest
  Relational Operator1 : RelationalOperator  Operator=>  OutDataTypeStr=boolean  RndMeth=Simplest
  O : Outport
  wires:
  Integrator/1 -> Relational Operator/2, Relational Operator1/2
  Logical Operator/1 -> O/1
  I/1 -> Compare To Zero/1
  Monostable/1 -> Integrator/2
  Constant/1 -> Integrator/1
  Fcn/1 -> Relational Operator/1
  Fcn1/1 -> Relational Operator1/1
  [ON] -> Logical Operator/4
  [alpha] -> Fcn/1, Fcn1/1
  Relational Operator/1 -> Logical Operator/1
  Compare To Zero/1 -> Monostable/1
  Relational Operator1/1 -> Logical Operator/2
  [CLK] -> Logical Operator/3

== system ModiOmkar_19EE30018_model/Gate Drive/Pulse Trafo #1/Subsystem ==
  D2 : powerlib/Power Electronics/Diode  Ron=0.001  Lon=0  Vf=0.7  IC=0  UseSnubber=off  Rs=inf  Cs=0  Measurements=off
  Data Type Conversion1 : DataTypeConversion  OutDataTypeStr=boolean
  R (for simulation) : powerlib/Elements/Series RLC Branch  LConnTagsString=__new0  RConnTagsString=__new0  BranchType=R  Resistance=100000  Inductance=60e-3  SetiL0=off  InitialCurrent=0  Capacitance=1e-6  Setx0=off  InitialVoltage=0  Measurements=None
  Relay1 : Relay  OnSwitchValue=0.36  OffSwitchValue=0.2
  Rg : powerlib/Elements/Series RLC Branch  LConnTagsString=__new0  RConnTagsString=__new0  BranchType=R  Resistance=20  Inductance=60e-3  SetiL0=off  InitialCurrent=0  Capacitance=1e-6  Setx0=off  InitialVoltage=0  Measurements=None
  Rgk : powerlib/Elements/Series RLC Branch  LConnTagsString=__new0  RConnTagsString=__new0  BranchType=R  Resistance=10  Inductance=60e-3  SetiL0=off  InitialCurrent=0  Capacitance=1e-6  Setx0=off  InitialVoltage=0  Measurements=None
  V_gk : powerlib/Measurements/Voltage Measurement  PhasorSimulation=off  OutputType=Complex  PSBequivalent=0
  +ve : PMIOPort  Side=Left
  -ve : PMIOPort  Port=2  Side=Left
  O : Outport
  wires:
  V_gk/1 -> Relay1/1
  Data Type Conversion1/1 -> O/1
  Relay1/1 -> Data Type Conversion1/1
  connections:
  D2/RConn1 -- V_gk/LConn1 -- Rgk/RConn1
  R (for simulation)/RConn1 -- D2/LConn1 -- Rg/LConn1
  +ve/RConn1 -- Rg/RConn1
  -ve/RConn1 -- R (for simulation)/LConn1 -- Rgk/LConn1 -- V_gk/LConn2

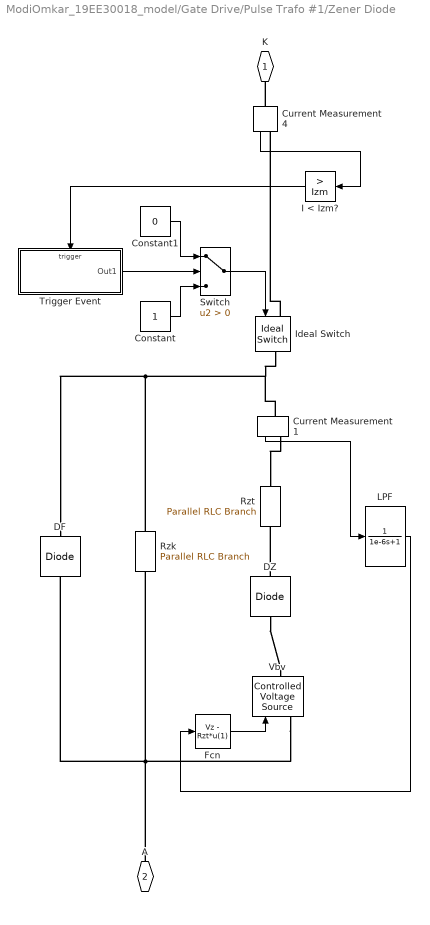
== system ModiOmkar_19EE30018_model/Gate Drive/Pulse Trafo #1/Zener Diode ==
  Constant : Constant
  Constant1 : Constant  Value=0
  Current Measurement1 : powerlib/Measurements/Current Measurement  PhasorSimulation=off  OutputType=Complex  PSBequivalent=0
  Current Measurement4 : powerlib/Measurements/Current Measurement  PhasorSimulation=off  OutputType=Complex  PSBequivalent=0
  DF : powerlib/Power Electronics/Diode  Ron=Ron  Lon=0  Vf=Vf  IC=0  UseSnubber=off  Rs=1000  Cs=0  Measurements=off
  DZ : powerlib/Power Electronics/Diode  Ron=1e-6  Lon=0  Vf=0  IC=0  UseSnubber=off  Rs=100  Cs=inf  Measurements=off
  Fcn : Fcn  Expr=Vz - Rzt*u(1)
  I < Izm? : simulink/Logic and Bit Operations/Compare To Constant  relop=>  const=Izm  OutDataTypeStr=boolean
  Ideal Switch : powerlib/Power Electronics/Ideal Switch  Ron=0.001  Lon=0  IC=1  Rs=1e5  Cs=0  Measurements=off
  LPF : TransferFcn  Denominator=[1e-6 1]
  Rzk : powerlib/Elements/Parallel RLC Branch  LConnTagsString=a  RConnTagsString=__new0  BranchType=R  Resistance=Rzk  Inductance=1.0  SetiL0=off  InitialCurrent=0  Capacitance=1e-5  Setx0=off  InitialVoltage=0  Measurements=None
  Rzt : powerlib/Elements/Parallel RLC Branch  LConnTagsString=a  RConnTagsString=__new0  BranchType=R  Resistance=Rzt  Inductance=1.0  SetiL0=off  InitialCurrent=0  Capacitance=1e-5  Setx0=off  InitialVoltage=0  Measurements=None
  Switch : Switch  Criteria=u2 > Threshold
  Trigger Event : Subsystem  TreatAsAtomicUnit=on
  Vbv : powerlib/Electrical Sources/Controlled Voltage Source  Initialize=off  Source_Type=DC  Amplitude=0  Phase=0  Frequency=0  Measurements=None
  K : PMIOPort  Side=Left
  A : PMIOPort  Port=2  Side=Right
  wires:
  Fcn/1 -> Vbv/1
  Current Measurement4/1 -> I < Izm?/1
  Current Measurement1/1 -> LPF/1
  LPF/1 -> Fcn/1
  I < Izm?/1 -> Trigger Event/Trigger
  Switch/1 -> Ideal Switch/1
  Trigger Event/1(Out1) -> Switch/2
  Constant/1 -> Switch/3
  Constant1/1 -> Switch/1
  connections:
  DZ/RConn1 -- Vbv/RConn1
  Current Measurement4/LConn1 -- K/RConn1
  DZ/LConn1 -- Rzt/LConn1
  Current Measurement1/RConn1 -- Rzt/RConn1
  Rzk/RConn1 -- Current Measurement1/LConn1 -- Ideal Switch/RConn1 -- DF/RConn1
  Ideal Switch/LConn1 -- Current Measurement4/RConn1
  A/RConn1 -- DF/LConn1 -- Rzk/LConn1 -- Vbv/LConn1

== system ModiOmkar_19EE30018_model/Gate Drive/Pulse Trafo #2/Subsystem ==
  D2 : powerlib/Power Electronics/Diode  Ron=0.001  Lon=0  Vf=0.7  IC=0  UseSnubber=off  Rs=inf  Cs=0  Measurements=off
  Data Type Conversion1 : DataTypeConversion  OutDataTypeStr=boolean
  R (for simulation) : powerlib/Elements/Series RLC Branch  LConnTagsString=__new0  RConnTagsString=__new0  BranchType=R  Resistance=100000  Inductance=60e-3  SetiL0=off  InitialCurrent=0  Capacitance=1e-6  Setx0=off  InitialVoltage=0  Measurements=None
  Relay1 : Relay  OnSwitchValue=0.36  OffSwitchValue=0.2
  Rg : powerlib/Elements/Series RLC Branch  LConnTagsString=__new0  RConnTagsString=__new0  BranchType=R  Resistance=20  Inductance=60e-3  SetiL0=off  InitialCurrent=0  Capacitance=1e-6  Setx0=off  InitialVoltage=0  Measurements=None
  Rgk : powerlib/Elements/Series RLC Branch  LConnTagsString=__new0  RConnTagsString=__new0  BranchType=R  Resistance=10  Inductance=60e-3  SetiL0=off  InitialCurrent=0  Capacitance=1e-6  Setx0=off  InitialVoltage=0  Measurements=None
  V_gk : powerlib/Measurements/Voltage Measurement  PhasorSimulation=off  OutputType=Complex  PSBequivalent=0
  +ve : PMIOPort  Side=Left
  -ve : PMIOPort  Port=2  Side=Left
  O : Outport
  wires:
  Relay1/1 -> Data Type Conversion1/1
  Data Type Conversion1/1 -> O/1
  V_gk/1 -> Relay1/1
  connections:
  V_gk/LConn2 -- Rgk/LConn1 -- R (for simulation)/LConn1 -- -ve/RConn1
  +ve/RConn1 -- Rg/RConn1
  Rg/LConn1 -- D2/LConn1 -- R (for simulation)/RConn1
  Rgk/RConn1 -- V_gk/LConn1 -- D2/RConn1

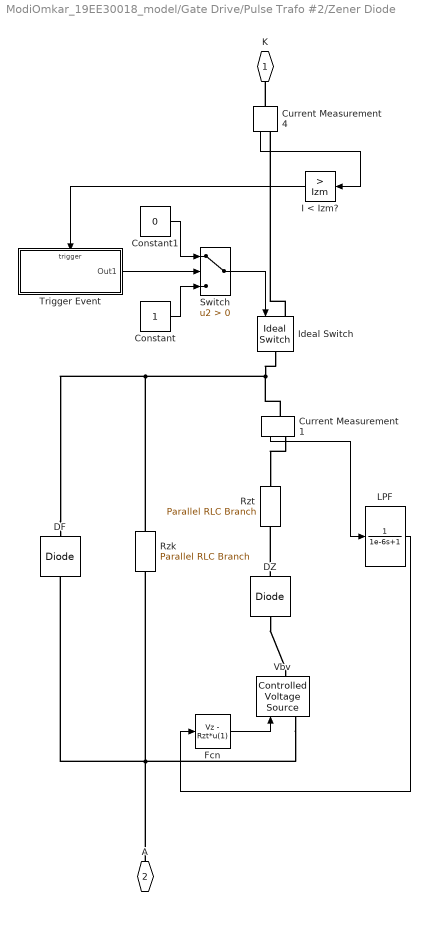
== system ModiOmkar_19EE30018_model/Gate Drive/Pulse Trafo #2/Zener Diode ==
  Constant : Constant
  Constant1 : Constant  Value=0
  Current Measurement1 : powerlib/Measurements/Current Measurement  PhasorSimulation=off  OutputType=Complex  PSBequivalent=0
  Current Measurement4 : powerlib/Measurements/Current Measurement  PhasorSimulation=off  OutputType=Complex  PSBequivalent=0
  DF : powerlib/Power Electronics/Diode  Ron=Ron  Lon=0  Vf=Vf  IC=0  UseSnubber=off  Rs=1000  Cs=0  Measurements=off
  DZ : powerlib/Power Electronics/Diode  Ron=1e-6  Lon=0  Vf=0  IC=0  UseSnubber=off  Rs=100  Cs=inf  Measurements=off
  Fcn : Fcn  Expr=Vz - Rzt*u(1)
  I < Izm? : simulink/Logic and Bit Operations/Compare To Constant  relop=>  const=Izm  OutDataTypeStr=boolean
  Ideal Switch : powerlib/Power Electronics/Ideal Switch  Ron=0.001  Lon=0  IC=1  Rs=1e5  Cs=0  Measurements=off
  LPF : TransferFcn  Denominator=[1e-6 1]
  Rzk : powerlib/Elements/Parallel RLC Branch  LConnTagsString=a  RConnTagsString=__new0  BranchType=R  Resistance=Rzk  Inductance=1.0  SetiL0=off  InitialCurrent=0  Capacitance=1e-5  Setx0=off  InitialVoltage=0  Measurements=None
  Rzt : powerlib/Elements/Parallel RLC Branch  LConnTagsString=a  RConnTagsString=__new0  BranchType=R  Resistance=Rzt  Inductance=1.0  SetiL0=off  InitialCurrent=0  Capacitance=1e-5  Setx0=off  InitialVoltage=0  Measurements=None
  Switch : Switch  Criteria=u2 > Threshold
  Trigger Event : Subsystem  TreatAsAtomicUnit=on
  Vbv : powerlib/Electrical Sources/Controlled Voltage Source  Initialize=off  Source_Type=DC  Amplitude=0  Phase=0  Frequency=0  Measurements=None
  K : PMIOPort  Side=Left
  A : PMIOPort  Port=2  Side=Right
  wires:
  Constant1/1 -> Switch/1
  Constant/1 -> Switch/3
  Trigger Event/1(Out1) -> Switch/2
  Switch/1 -> Ideal Switch/1
  I < Izm?/1 -> Trigger Event/Trigger
  LPF/1 -> Fcn/1
  Current Measurement1/1 -> LPF/1
  Current Measurement4/1 -> I < Izm?/1
  Fcn/1 -> Vbv/1
  connections:
  Vbv/LConn1 -- Rzk/LConn1 -- DF/LConn1 -- A/RConn1
  Ideal Switch/LConn1 -- Current Measurement4/RConn1
  DF/RConn1 -- Ideal Switch/RConn1 -- Current Measurement1/LConn1 -- Rzk/RConn1
  Current Measurement1/RConn1 -- Rzt/RConn1
  DZ/LConn1 -- Rzt/LConn1
  Current Measurement4/LConn1 -- K/RConn1
  DZ/RConn1 -- Vbv/RConn1

== system ModiOmkar_19EE30018_model/Gate Drive/Pulse Trafo #3/Subsystem ==
  D2 : powerlib/Power Electronics/Diode  Ron=0.001  Lon=0  Vf=0.7  IC=0  UseSnubber=off  Rs=inf  Cs=0  Measurements=off
  Data Type Conversion1 : DataTypeConversion  OutDataTypeStr=boolean
  R (for simulation) : powerlib/Elements/Series RLC Branch  LConnTagsString=__new0  RConnTagsString=__new0  BranchType=R  Resistance=100000  Inductance=60e-3  SetiL0=off  InitialCurrent=0  Capacitance=1e-6  Setx0=off  InitialVoltage=0  Measurements=None
  Relay1 : Relay  OnSwitchValue=0.36  OffSwitchValue=0.2
  Rg : powerlib/Elements/Series RLC Branch  LConnTagsString=__new0  RConnTagsString=__new0  BranchType=R  Resistance=20  Inductance=60e-3  SetiL0=off  InitialCurrent=0  Capacitance=1e-6  Setx0=off  InitialVoltage=0  Measurements=None
  Rgk : powerlib/Elements/Series RLC Branch  LConnTagsString=__new0  RConnTagsString=__new0  BranchType=R  Resistance=10  Inductance=60e-3  SetiL0=off  InitialCurrent=0  Capacitance=1e-6  Setx0=off  InitialVoltage=0  Measurements=None
  V_gk : powerlib/Measurements/Voltage Measurement  PhasorSimulation=off  OutputType=Complex  PSBequivalent=0
  +ve : PMIOPort  Side=Left
  -ve : PMIOPort  Port=2  Side=Left
  O : Outport
  wires:
  V_gk/1 -> Relay1/1
  Data Type Conversion1/1 -> O/1
  Relay1/1 -> Data Type Conversion1/1
  connections:
  D2/RConn1 -- V_gk/LConn1 -- Rgk/RConn1
  R (for simulation)/RConn1 -- D2/LConn1 -- Rg/LConn1
  +ve/RConn1 -- Rg/RConn1
  -ve/RConn1 -- R (for simulation)/LConn1 -- Rgk/LConn1 -- V_gk/LConn2

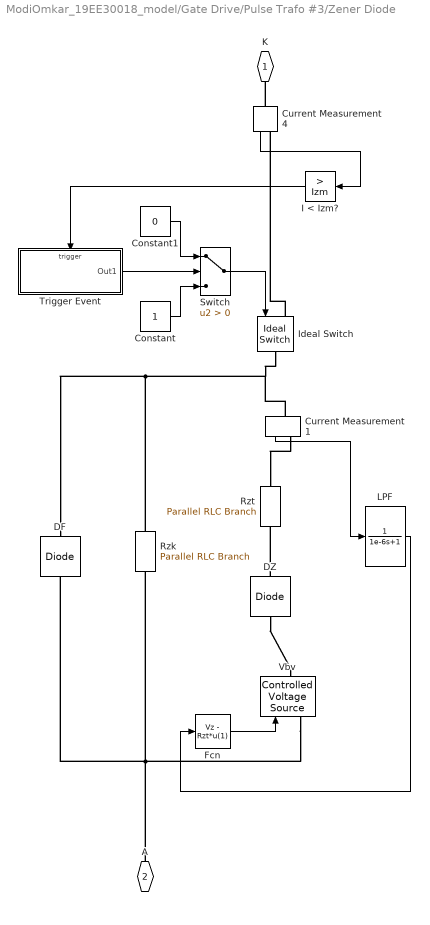
== system ModiOmkar_19EE30018_model/Gate Drive/Pulse Trafo #3/Zener Diode ==
  Constant : Constant
  Constant1 : Constant  Value=0
  Current Measurement1 : powerlib/Measurements/Current Measurement  PhasorSimulation=off  OutputType=Complex  PSBequivalent=0
  Current Measurement4 : powerlib/Measurements/Current Measurement  PhasorSimulation=off  OutputType=Complex  PSBequivalent=0
  DF : powerlib/Power Electronics/Diode  Ron=Ron  Lon=0  Vf=Vf  IC=0  UseSnubber=off  Rs=1000  Cs=0  Measurements=off
  DZ : powerlib/Power Electronics/Diode  Ron=1e-6  Lon=0  Vf=0  IC=0  UseSnubber=off  Rs=100  Cs=inf  Measurements=off
  Fcn : Fcn  Expr=Vz - Rzt*u(1)
  I < Izm? : simulink/Logic and Bit Operations/Compare To Constant  relop=>  const=Izm  OutDataTypeStr=boolean
  Ideal Switch : powerlib/Power Electronics/Ideal Switch  Ron=0.001  Lon=0  IC=1  Rs=1e5  Cs=0  Measurements=off
  LPF : TransferFcn  Denominator=[1e-6 1]
  Rzk : powerlib/Elements/Parallel RLC Branch  LConnTagsString=a  RConnTagsString=__new0  BranchType=R  Resistance=Rzk  Inductance=1.0  SetiL0=off  InitialCurrent=0  Capacitance=1e-5  Setx0=off  InitialVoltage=0  Measurements=None
  Rzt : powerlib/Elements/Parallel RLC Branch  LConnTagsString=a  RConnTagsString=__new0  BranchType=R  Resistance=Rzt  Inductance=1.0  SetiL0=off  InitialCurrent=0  Capacitance=1e-5  Setx0=off  InitialVoltage=0  Measurements=None
  Switch : Switch  Criteria=u2 > Threshold
  Trigger Event : Subsystem  TreatAsAtomicUnit=on
  Vbv : powerlib/Electrical Sources/Controlled Voltage Source  Initialize=off  Source_Type=DC  Amplitude=0  Phase=0  Frequency=0  Measurements=None
  K : PMIOPort  Side=Left
  A : PMIOPort  Port=2  Side=Right
  wires:
  Fcn/1 -> Vbv/1
  Current Measurement4/1 -> I < Izm?/1
  Current Measurement1/1 -> LPF/1
  LPF/1 -> Fcn/1
  I < Izm?/1 -> Trigger Event/Trigger
  Switch/1 -> Ideal Switch/1
  Trigger Event/1(Out1) -> Switch/2
  Constant/1 -> Switch/3
  Constant1/1 -> Switch/1
  connections:
  DZ/RConn1 -- Vbv/RConn1
  Current Measurement4/LConn1 -- K/RConn1
  DZ/LConn1 -- Rzt/LConn1
  Current Measurement1/RConn1 -- Rzt/RConn1
  Rzk/RConn1 -- Current Measurement1/LConn1 -- Ideal Switch/RConn1 -- DF/RConn1
  Ideal Switch/LConn1 -- Current Measurement4/RConn1
  A/RConn1 -- DF/LConn1 -- Rzk/LConn1 -- Vbv/LConn1

== system ModiOmkar_19EE30018_model/Gate Drive/Pulse Trafo #4/Subsystem ==
  D2 : powerlib/Power Electronics/Diode  Ron=0.001  Lon=0  Vf=0.7  IC=0  UseSnubber=off  Rs=inf  Cs=0  Measurements=off
  Data Type Conversion1 : DataTypeConversion  OutDataTypeStr=boolean
  R (for simulation) : powerlib/Elements/Series RLC Branch  LConnTagsString=__new0  RConnTagsString=__new0  BranchType=R  Resistance=100000  Inductance=60e-3  SetiL0=off  InitialCurrent=0  Capacitance=1e-6  Setx0=off  InitialVoltage=0  Measurements=None
  Relay1 : Relay  OnSwitchValue=0.36  OffSwitchValue=0.2
  Rg : powerlib/Elements/Series RLC Branch  LConnTagsString=__new0  RConnTagsString=__new0  BranchType=R  Resistance=20  Inductance=60e-3  SetiL0=off  InitialCurrent=0  Capacitance=1e-6  Setx0=off  InitialVoltage=0  Measurements=None
  Rgk : powerlib/Elements/Series RLC Branch  LConnTagsString=__new0  RConnTagsString=__new0  BranchType=R  Resistance=10  Inductance=60e-3  SetiL0=off  InitialCurrent=0  Capacitance=1e-6  Setx0=off  InitialVoltage=0  Measurements=None
  V_gk : powerlib/Measurements/Voltage Measurement  PhasorSimulation=off  OutputType=Complex  PSBequivalent=0
  +ve : PMIOPort  Side=Left
  -ve : PMIOPort  Port=2  Side=Left
  O : Outport
  wires:
  Relay1/1 -> Data Type Conversion1/1
  Data Type Conversion1/1 -> O/1
  V_gk/1 -> Relay1/1
  connections:
  V_gk/LConn2 -- Rgk/LConn1 -- R (for simulation)/LConn1 -- -ve/RConn1
  +ve/RConn1 -- Rg/RConn1
  Rg/LConn1 -- D2/LConn1 -- R (for simulation)/RConn1
  Rgk/RConn1 -- V_gk/LConn1 -- D2/RConn1

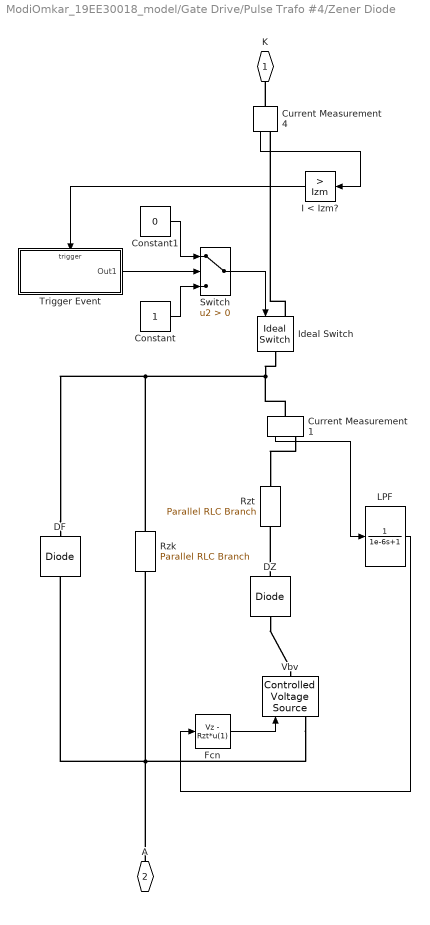
== system ModiOmkar_19EE30018_model/Gate Drive/Pulse Trafo #4/Zener Diode ==
  Constant : Constant
  Constant1 : Constant  Value=0
  Current Measurement1 : powerlib/Measurements/Current Measurement  PhasorSimulation=off  OutputType=Complex  PSBequivalent=0
  Current Measurement4 : powerlib/Measurements/Current Measurement  PhasorSimulation=off  OutputType=Complex  PSBequivalent=0
  DF : powerlib/Power Electronics/Diode  Ron=Ron  Lon=0  Vf=Vf  IC=0  UseSnubber=off  Rs=1000  Cs=0  Measurements=off
  DZ : powerlib/Power Electronics/Diode  Ron=1e-6  Lon=0  Vf=0  IC=0  UseSnubber=off  Rs=100  Cs=inf  Measurements=off
  Fcn : Fcn  Expr=Vz - Rzt*u(1)
  I < Izm? : simulink/Logic and Bit Operations/Compare To Constant  relop=>  const=Izm  OutDataTypeStr=boolean
  Ideal Switch : powerlib/Power Electronics/Ideal Switch  Ron=0.001  Lon=0  IC=1  Rs=1e5  Cs=0  Measurements=off
  LPF : TransferFcn  Denominator=[1e-6 1]
  Rzk : powerlib/Elements/Parallel RLC Branch  LConnTagsString=a  RConnTagsString=__new0  BranchType=R  Resistance=Rzk  Inductance=1.0  SetiL0=off  InitialCurrent=0  Capacitance=1e-5  Setx0=off  InitialVoltage=0  Measurements=None
  Rzt : powerlib/Elements/Parallel RLC Branch  LConnTagsString=a  RConnTagsString=__new0  BranchType=R  Resistance=Rzt  Inductance=1.0  SetiL0=off  InitialCurrent=0  Capacitance=1e-5  Setx0=off  InitialVoltage=0  Measurements=None
  Switch : Switch  Criteria=u2 > Threshold
  Trigger Event : Subsystem  TreatAsAtomicUnit=on
  Vbv : powerlib/Electrical Sources/Controlled Voltage Source  Initialize=off  Source_Type=DC  Amplitude=0  Phase=0  Frequency=0  Measurements=None
  K : PMIOPort  Side=Left
  A : PMIOPort  Port=2  Side=Right
  wires:
  Constant1/1 -> Switch/1
  Constant/1 -> Switch/3
  Trigger Event/1(Out1) -> Switch/2
  Switch/1 -> Ideal Switch/1
  I < Izm?/1 -> Trigger Event/Trigger
  LPF/1 -> Fcn/1
  Current Measurement1/1 -> LPF/1
  Current Measurement4/1 -> I < Izm?/1
  Fcn/1 -> Vbv/1
  connections:
  Vbv/LConn1 -- Rzk/LConn1 -- DF/LConn1 -- A/RConn1
  Ideal Switch/LConn1 -- Current Measurement4/RConn1
  DF/RConn1 -- Ideal Switch/RConn1 -- Current Measurement1/LConn1 -- Rzk/RConn1
  Current Measurement1/RConn1 -- Rzt/RConn1
  DZ/LConn1 -- Rzt/LConn1
  Current Measurement4/LConn1 -- K/RConn1
  DZ/RConn1 -- Vbv/RConn1
